simulink model "svc_go_d"  (R2023a)
settings: Solver=FixedStepDiscrete  StartTime=0.0  StopTime=2.0  FixedStep=Ts  RelTol=1e-3
InitFcn:
  | svc_go_init
values from neighbouring files (symbols this model uses):
  ki = [ki1 ki2]    [est_model_paras.m]    (also in svc_go_init.m = 2.96*Rs/sqrt(2)/N/Ts)
  kp = (3*Ld./N/Ts-Rs)/Lq/Iq    [est_model_paras.m]    (also in svc_go_init.m = -0.01944)
  Ld = 0.000891    [est_model_paras.m]    (also in svc_go_init.m = 0.00026)
  Lq = 0.000891    [est_model_paras.m]    (also in svc_go_init.m = 0.000636)
  phi_r = 0.012    [est_model_paras.m]    (also in svc_go_init.m = 0.078)
  Rs = 0.503    [est_model_paras.m]    (also in svc_go_init.m = 0.021)
  Ts = 1/8000    (= 0.000125)    [est_model_paras.m]    (also in svc_go_init.m)
  We = 2*pi*100    (= 628.318530718)    [est_model_paras.m]    (also in svc_go_init.m)
undefined symbols (not defined in the file or in its folder): DiscIntNeverNeededParam
libraries: slpidlib x3
settings Model: Creator=LG-PC  LastModifiedBy=洲
settings SolverCC: AlgebraicLoopSolver=TrustRegion
settings DataIOCC: ReturnWorkspaceOutputs=off
settings DebuggingCC: UnconnectedInputMsg=warning  UnconnectedOutputMsg=warning  UnconnectedLineMsg=warning  ArithmeticOperatorsInVariantConditions=warning
settings ModelReferenceCC: EnableRefExpFcnMdlSchedulingChecks=on
settings SFSimCC: SimUseLocalCustomCode=off  CustomCodeUndefinedFunction=UseInterfaceOnly
settings RTWCC: RTWUseLocalCustomCode=off

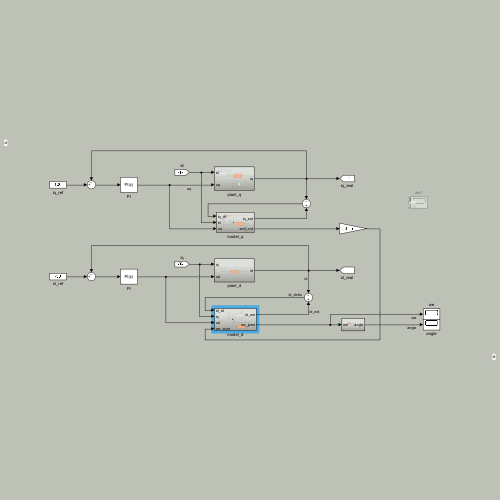
[thumbnail: Simulink's stored preview of the top-level diagram]
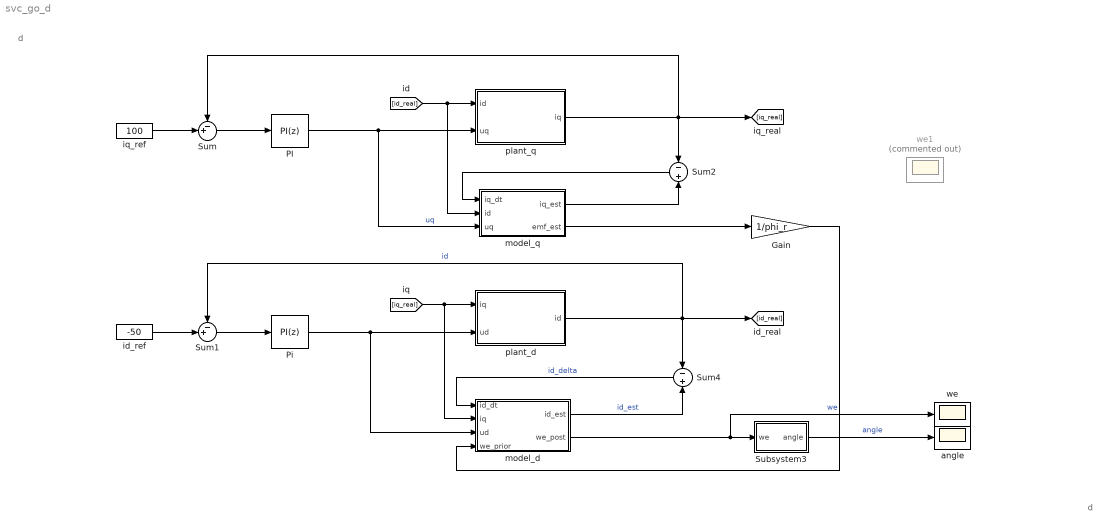
== system svc_go_d ==
  note: d
  note: d
  Gain : Gain  Gain=1/phi_r
  PI : slpidlib/PID Controller  Controller=PI  Form=Parallel  TimeDomain=Discrete-time  UseExternalTs=off  SampleTime=-1  IntegratorMethod=Forward Euler  FilterMethod=Forward Euler  ControllerParametersSource=internal  P=1  I=50  UseKiTs=off  D=0  N=100  UseFilter=on  TunerSelectOption=Transfer Function Based (PID Tuner App)  InitialConditionSource=internal  InitialConditionForIntegrator=0  InitialConditionForFilter=0  DifferentiatorICPrevScaledInput=0  ExternalReset=none  TrackingMode=off  Kt=1  LimitOutput=off  SatLimitsSource=internal  UpperSaturationLimit=inf  LowerSaturationLimit=-inf  LinearizeAsGain=on  AntiWindupMode=none  Kb=1  LimitIntegrator=off  UpperIntegratorSaturationLimit=inf  LowerIntegratorSaturationLimit=-inf  POutMin=[]  POutMax=[]  IOutMin=[]  IOutMax=[]  DOutMin=[]  DOutMax=[]  NOutMin=[]  NOutMax=[]  SumOutMin=[]  SumOutMax=[]  SaturationOutMin=[]  SaturationOutMax=[]  PParamMin=[]  PParamMax=[]  IParamMin=[]  IParamMax=[]  DParamMin=[]  DParamMax=[]  NParamMin=[]  NParamMax=[]  KbParamMin=[]  KbParamMax=[]  KtParamMin=[]  KtParamMax=[]  KbOutMin=[]  KbOutMax=[]  KtOutMin=[]  KtOutMax=[]  IntegratorOutMin=[]  IntegratorOutMax=[]  FilterOutMin=[]  FilterOutMax=[]  SumI1OutMin=[]  SumI1OutMax=[]  SumI2OutMin=[]  SumI2OutMax=[]  SumI3OutMin=[]  SumI3OutMax=[]  SumI4OutMin=[]  SumI4OutMax=[]  SumDOutMin=[]  SumDOutMax=[]  DifferentiatorOutMin=[]  DifferentiatorOutMax=[]  FilterDiffOutCoefMin=[]  FilterDiffOutCoefMax=[]  ReciprocalOutMin=[]  ReciprocalOutMax=[]  SumDenOutMin=[]  SumDenOutMax=[]  SumNumOutMin=[]  SumNumOutMax=[]  DivideOutMin=[]  DivideOutMax=[]  UdiffTsProdOutMin=[]  UdiffTsProdOutMax=[]  NTsProdOutMin=[]  NTsProdOutMax=[]  UintegralTsProdOutMin=[]  UintegralTsProdOutMax=[]  UngainTsProdOutMin=[]  UngainTsProdOutMax=[]  ClampingZeroOutDataTypeStr=Inherit: Inherit via back propagation  ClampingZeroOutMin=[]  ClampingZeroOutMax=[]  FilterDenConstantOutDataTypeStr=Inherit: Inherit via back propagation  FilterDenConstantOutMin=[]  FilterDenConstantOutMax=[]  PCopyOutDataTypeStr=Inherit: Inherit via back propagation  PCopyOutMin=[]  PCopyOutMax=[]  NCopyOutDataTypeStr=Inherit: Inherit via back propagation  NCopyOutMin=[]  NCopyOutMax=[]  IntegratorContinuousStateAttributes=''  IntegratorStateMustResolveToSignalObject=off  IntegratorRTWStateStorageClass=Auto  FilterContinuousStateAttributes=''  FilterStateMustResolveToSignalObject=off  FilterRTWStateStorageClass=Auto  ParallelPVariant=InternalParameters  IdealPVariant=Disabled  IVariant=InternalParameters  DVariant=Disabled  IntegratorVariant=Discrete  SatVariant=Disabled  AWVariant=Passthrough  PCopyVariant=Disabled  TRVariant=Disabled  FdbkBlocksVariant=Forward  IdealPFdbkVariant=Disabled  SatFdbkVariant=Disabled  DerivativeFilterVariant=Disabled  NVariant=Disabled  NCopyVariant=Disabled_SignalSpec  FilterICVariant=Disabled  IntegratorICVariant=InternalICs  ExternalResetVariant=Disabled  TRSumVariant=Passthrough  SumFdbkVariant=Disabled  SumVariant=Sum_PI  TsampFilterVariant=InternalTs  TsampNgainVariant=Passthrough  TsampIntegralVariant=Disabled_SignalSpec  ExternalSaturationOutDataTypeStr=Inherit: Same as second input
  Pi : slpidlib/PID Controller  Controller=PI  Form=Parallel  TimeDomain=Discrete-time  UseExternalTs=off  SampleTime=-1  IntegratorMethod=Forward Euler  FilterMethod=Forward Euler  ControllerParametersSource=internal  P=1  I=50  UseKiTs=off  D=0  N=100  UseFilter=on  TunerSelectOption=Transfer Function Based (PID Tuner App)  InitialConditionSource=internal  InitialConditionForIntegrator=0  InitialConditionForFilter=0  DifferentiatorICPrevScaledInput=0  ExternalReset=none  TrackingMode=off  Kt=1  LimitOutput=off  SatLimitsSource=internal  UpperSaturationLimit=inf  LowerSaturationLimit=-inf  LinearizeAsGain=on  AntiWindupMode=none  Kb=1  LimitIntegrator=off  UpperIntegratorSaturationLimit=inf  LowerIntegratorSaturationLimit=-inf  POutMin=[]  POutMax=[]  IOutMin=[]  IOutMax=[]  DOutMin=[]  DOutMax=[]  NOutMin=[]  NOutMax=[]  SumOutMin=[]  SumOutMax=[]  SaturationOutMin=[]  SaturationOutMax=[]  PParamMin=[]  PParamMax=[]  IParamMin=[]  IParamMax=[]  DParamMin=[]  DParamMax=[]  NParamMin=[]  NParamMax=[]  KbParamMin=[]  KbParamMax=[]  KtParamMin=[]  KtParamMax=[]  KbOutMin=[]  KbOutMax=[]  KtOutMin=[]  KtOutMax=[]  IntegratorOutMin=[]  IntegratorOutMax=[]  FilterOutMin=[]  FilterOutMax=[]  SumI1OutMin=[]  SumI1OutMax=[]  SumI2OutMin=[]  SumI2OutMax=[]  SumI3OutMin=[]  SumI3OutMax=[]  SumI4OutMin=[]  SumI4OutMax=[]  SumDOutMin=[]  SumDOutMax=[]  DifferentiatorOutMin=[]  DifferentiatorOutMax=[]  FilterDiffOutCoefMin=[]  FilterDiffOutCoefMax=[]  ReciprocalOutMin=[]  ReciprocalOutMax=[]  SumDenOutMin=[]  SumDenOutMax=[]  SumNumOutMin=[]  SumNumOutMax=[]  DivideOutMin=[]  DivideOutMax=[]  UdiffTsProdOutMin=[]  UdiffTsProdOutMax=[]  NTsProdOutMin=[]  NTsProdOutMax=[]  UintegralTsProdOutMin=[]  UintegralTsProdOutMax=[]  UngainTsProdOutMin=[]  UngainTsProdOutMax=[]  ClampingZeroOutDataTypeStr=Inherit: Inherit via back propagation  ClampingZeroOutMin=[]  ClampingZeroOutMax=[]  FilterDenConstantOutDataTypeStr=Inherit: Inherit via back propagation  FilterDenConstantOutMin=[]  FilterDenConstantOutMax=[]  PCopyOutDataTypeStr=Inherit: Inherit via back propagation  PCopyOutMin=[]  PCopyOutMax=[]  NCopyOutDataTypeStr=Inherit: Inherit via back propagation  NCopyOutMin=[]  NCopyOutMax=[]  IntegratorContinuousStateAttributes=''  IntegratorStateMustResolveToSignalObject=off  IntegratorRTWStateStorageClass=Auto  FilterContinuousStateAttributes=''  FilterStateMustResolveToSignalObject=off  FilterRTWStateStorageClass=Auto  ParallelPVariant=InternalParameters  IdealPVariant=Disabled  IVariant=InternalParameters  DVariant=Disabled  IntegratorVariant=Discrete  SatVariant=Disabled  AWVariant=Passthrough  PCopyVariant=Disabled  TRVariant=Disabled  FdbkBlocksVariant=Forward  IdealPFdbkVariant=Disabled  SatFdbkVariant=Disabled  DerivativeFilterVariant=Disabled  NVariant=Disabled  NCopyVariant=Disabled_SignalSpec  FilterICVariant=Disabled  IntegratorICVariant=InternalICs  ExternalResetVariant=Disabled  TRSumVariant=Passthrough  SumFdbkVariant=Disabled  SumVariant=Sum_PI  TsampFilterVariant=InternalTs  TsampNgainVariant=Passthrough  TsampIntegralVariant=Disabled_SignalSpec  ExternalSaturationOutDataTypeStr=Inherit: Same as second input
  Subsystem3 : Subsystem
  Sum : Sum  Inputs=-+|
  Sum1 : Sum  Inputs=-+|
  Sum2 : Sum  Inputs=-+
  Sum4 : Sum  Inputs=-+
  angle : Scope
  id_ref : Constant  Value=-50
  iq_ref : Constant  Value=100
  model_d : Subsystem
  model_q : Subsystem
  plant_d : Subsystem
  plant_q : Subsystem
  we : Scope
  we1 : Scope  Commented=on  NumInputPorts=2
  wires:
  PI/1 -> plant_q/2(uq), model_q/3(uq)  "uq"
  Sum/1 -> PI/1
  Sum2/1 -> model_q/1(iq_dt)
  model_q/1(iq_est) -> Sum2/2
  plant_q/1(iq) -> Sum/1, [iq_real], Sum2/1
  [id_real] -> model_q/2(id), plant_q/1(id)
  iq_ref/1 -> Sum/2
  id_ref/1 -> Sum1/2
  Sum1/1 -> Pi/1
  Pi/1 -> model_d/3(ud), plant_d/2(ud)
  plant_d/1(id) -> Sum1/1, Sum4/1, [id_real]  "id"
  [iq_real] -> plant_d/1(iq), model_d/2(iq)
  Sum4/1 -> model_d/1(id_dt)  "id_delta"
  model_d/1(id_est) -> Sum4/2  "id_est"
  Gain/1 -> model_d/4(we_prior)
  model_q/2(emf_est) -> Gain/1
  model_d/2(we_post) -> we/1, Subsystem3/1(we)  "we"
  Subsystem3/1(angle) -> angle/1  "angle"

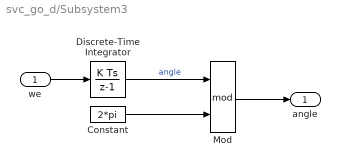
== system svc_go_d/Subsystem3 ==
  we : Inport
  Constant : Constant  Value=2*pi
  Discrete-Time Integrator : DiscreteIntegrator  SampleTime=-1  ICPrevOutput=DiscIntNeverNeededParam  ICPrevScaledInput=DiscIntNeverNeededParam
  Mod : Math  Operator=mod  SignedPower=on
  angle : Outport  VectorParamsAs1DForOutWhenUnconnected=off
  wires:
  Constant/1 -> Mod/2
  we/1 -> Discrete-Time Integrator/1
  Mod/1 -> angle/1
  Discrete-Time Integrator/1 -> Mod/1  "angle"

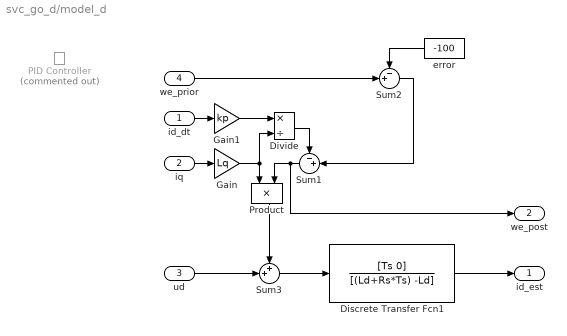
== system svc_go_d/model_d ==
  id_dt : Inport
  iq : Inport  Port=2
  ud : Inport  Port=3
  we_prior : Inport  Port=4
  Discrete Transfer Fcn1 : DiscreteTransferFcn  Numerator=[Ts 0]  Denominator=[(Ld+Rs*Ts) -Ld]
  Divide : Product  Inputs=*/
  Gain : Gain  Gain=Lq
  Gain1 : Gain  Gain=kp
  PID Controller : slpidlib/PID Controller  Commented=on  Controller=PI  Form=Parallel  TimeDomain=Continuous-time  UseExternalTs=off  SampleTime=-1  IntegratorMethod=Forward Euler  FilterMethod=Forward Euler  ControllerParametersSource=internal  P=100  I=0  UseKiTs=off  D=0  N=100  UseFilter=on  TunerSelectOption=Transfer Function Based (PID Tuner App)  InitialConditionSource=internal  InitialConditionForIntegrator=0  InitialConditionForFilter=0  DifferentiatorICPrevScaledInput=0  ExternalReset=none  TrackingMode=off  Kt=1  LimitOutput=off  SatLimitsSource=internal  UpperSaturationLimit=inf  LowerSaturationLimit=-inf  LinearizeAsGain=on  AntiWindupMode=none  Kb=1  LimitIntegrator=off  UpperIntegratorSaturationLimit=inf  LowerIntegratorSaturationLimit=-inf  POutMin=[]  POutMax=[]  IOutMin=[]  IOutMax=[]  DOutMin=[]  DOutMax=[]  NOutMin=[]  NOutMax=[]  SumOutMin=[]  SumOutMax=[]  SaturationOutMin=[]  SaturationOutMax=[]  PParamMin=[]  PParamMax=[]  IParamMin=[]  IParamMax=[]  DParamMin=[]  DParamMax=[]  NParamMin=[]  NParamMax=[]  KbParamMin=[]  KbParamMax=[]  KtParamMin=[]  KtParamMax=[]  KbOutMin=[]  KbOutMax=[]  KtOutMin=[]  KtOutMax=[]  IntegratorOutMin=[]  IntegratorOutMax=[]  FilterOutMin=[]  FilterOutMax=[]  SumI1OutMin=[]  SumI1OutMax=[]  SumI2OutMin=[]  SumI2OutMax=[]  SumI3OutMin=[]  SumI3OutMax=[]  SumI4OutMin=[]  SumI4OutMax=[]  SumDOutMin=[]  SumDOutMax=[]  DifferentiatorOutMin=[]  DifferentiatorOutMax=[]  FilterDiffOutCoefMin=[]  FilterDiffOutCoefMax=[]  ReciprocalOutMin=[]  ReciprocalOutMax=[]  SumDenOutMin=[]  SumDenOutMax=[]  SumNumOutMin=[]  SumNumOutMax=[]  DivideOutMin=[]  DivideOutMax=[]  UdiffTsProdOutMin=[]  UdiffTsProdOutMax=[]  NTsProdOutMin=[]  NTsProdOutMax=[]  UintegralTsProdOutMin=[]  UintegralTsProdOutMax=[]  UngainTsProdOutMin=[]  UngainTsProdOutMax=[]  ClampingZeroOutDataTypeStr=Inherit: Inherit via back propagation  ClampingZeroOutMin=[]  ClampingZeroOutMax=[]  FilterDenConstantOutDataTypeStr=Inherit: Inherit via back propagation  FilterDenConstantOutMin=[]  FilterDenConstantOutMax=[]  PCopyOutDataTypeStr=Inherit: Inherit via back propagation  PCopyOutMin=[]  PCopyOutMax=[]  NCopyOutDataTypeStr=Inherit: Inherit via back propagation  NCopyOutMin=[]  NCopyOutMax=[]  IntegratorContinuousStateAttributes=''  IntegratorStateMustResolveToSignalObject=off  IntegratorRTWStateStorageClass=Auto  FilterContinuousStateAttributes=''  FilterStateMustResolveToSignalObject=off  FilterRTWStateStorageClass=Auto  ParallelPVariant=InternalParameters  IdealPVariant=Disabled  IVariant=InternalParameters  DVariant=Disabled  IntegratorVariant=Continuous  SatVariant=Disabled  AWVariant=Passthrough  PCopyVariant=Disabled  TRVariant=Disabled  FdbkBlocksVariant=Forward  IdealPFdbkVariant=Disabled  SatFdbkVariant=Disabled  DerivativeFilterVariant=Disabled  NVariant=Disabled  NCopyVariant=Disabled_SignalSpec  FilterICVariant=Disabled  IntegratorICVariant=InternalICs  ExternalResetVariant=Disabled  TRSumVariant=Passthrough  SumFdbkVariant=Disabled  SumVariant=Sum_PI  TsampFilterVariant=InternalTs  TsampNgainVariant=Passthrough  TsampIntegralVariant=Disabled_SignalSpec  ExternalSaturationOutDataTypeStr=Inherit: Same as second input
  Product : Product
  Sum1 : Sum  Inputs=-+|
  Sum2 : Sum  Inputs=-+|
  Sum3 : Sum  Inputs=++|
  error : Constant  Value=-100
  id_est : Outport  VectorParamsAs1DForOutWhenUnconnected=off
  we_post : Outport  Port=2  VectorParamsAs1DForOutWhenUnconnected=off
  wires:
  iq/1 -> Gain/1
  ud/1 -> Sum3/2
  Sum3/1 -> Discrete Transfer Fcn1/1
  Gain/1 -> Divide/2, Product/1
  Product/1 -> Sum3/1
  Sum1/1 -> we_post/1, Product/2
  we_prior/1 -> Sum2/2
  error/1 -> Sum2/1
  Sum2/1 -> Sum1/2
  Discrete Transfer Fcn1/1 -> id_est/1
  id_dt/1 -> Gain1/1
  Divide/1 -> Sum1/1
  Gain1/1 -> Divide/1

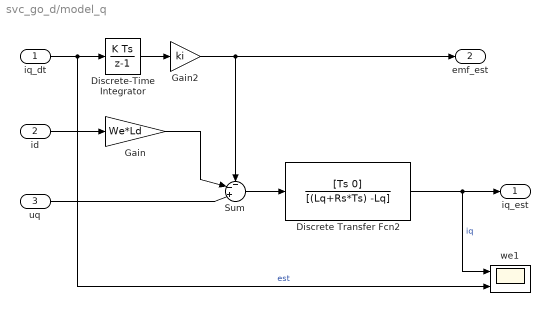
== system svc_go_d/model_q ==
  iq_dt : Inport
  id : Inport  Port=2
  uq : Inport  Port=3
  Discrete Transfer Fcn2 : DiscreteTransferFcn  Numerator=[Ts 0]  Denominator=[(Lq+Rs*Ts) -Lq]
  Discrete-Time Integrator : DiscreteIntegrator  SampleTime=-1  ICPrevOutput=DiscIntNeverNeededParam  ICPrevScaledInput=DiscIntNeverNeededParam
  Gain : Gain  Gain=We*Ld
  Gain2 : Gain  Gain=ki
  Sum : Sum  Inputs=--+|
  we1 : Scope  NumInputPorts=2
  iq_est : Outport  VectorParamsAs1DForOutWhenUnconnected=off
  emf_est : Outport  Port=2  VectorParamsAs1DForOutWhenUnconnected=off
  wires:
  iq_dt/1 -> we1/2, Discrete-Time Integrator/1  "est"
  Discrete-Time Integrator/1 -> Gain2/1
  Gain/1 -> Sum/2
  uq/1 -> Sum/3
  Sum/1 -> Discrete Transfer Fcn2/1
  Gain2/1 -> emf_est/1, Sum/1
  Discrete Transfer Fcn2/1 -> we1/1, iq_est/1  "iq"
  id/1 -> Gain/1

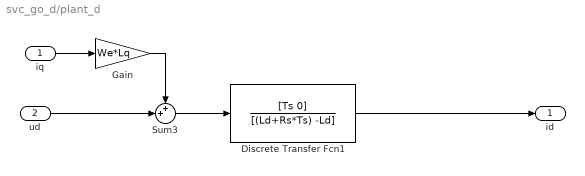
== system svc_go_d/plant_d ==
  iq : Inport
  ud : Inport  Port=2
  Discrete Transfer Fcn1 : DiscreteTransferFcn  Numerator=[Ts 0]  Denominator=[(Ld+Rs*Ts) -Ld]
  Gain : Gain  Gain=We*Lq
  Sum3 : Sum  Inputs=++|
  id : Outport  VectorParamsAs1DForOutWhenUnconnected=off
  wires:
  iq/1 -> Gain/1
  ud/1 -> Sum3/2
  Sum3/1 -> Discrete Transfer Fcn1/1
  Gain/1 -> Sum3/1
  Discrete Transfer Fcn1/1 -> id/1

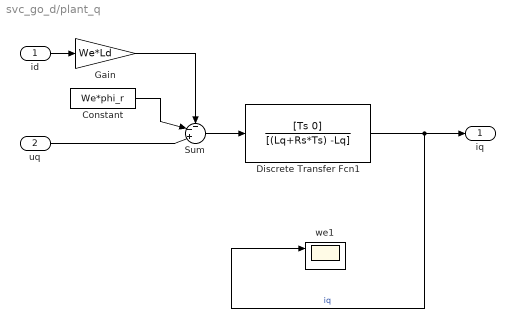
== system svc_go_d/plant_q ==
  id : Inport
  uq : Inport  Port=2
  Constant : Constant  Value=We*phi_r
  Discrete Transfer Fcn1 : DiscreteTransferFcn  Numerator=[Ts 0]  Denominator=[(Lq+Rs*Ts) -Lq]
  Gain : Gain  Gain=We*Ld
  Sum : Sum  Inputs=--+|
  we1 : Scope  NumInputPorts=2
  iq : Outport  VectorParamsAs1DForOutWhenUnconnected=off
  wires:
  id/1 -> Gain/1
  Discrete Transfer Fcn1/1 -> we1/1, iq/1  "iq"
  Sum/1 -> Discrete Transfer Fcn1/1
  uq/1 -> Sum/3
  Gain/1 -> Sum/1
  Constant/1 -> Sum/2
